simulink model "Copy_of_piddd"  (R2015b)
settings: Solver=VariableStepAuto  StartTime=0.0  StopTime=10.0  RelTol=1e-3
settings Model: Creator=ECPKn  LastModifiedBy=li

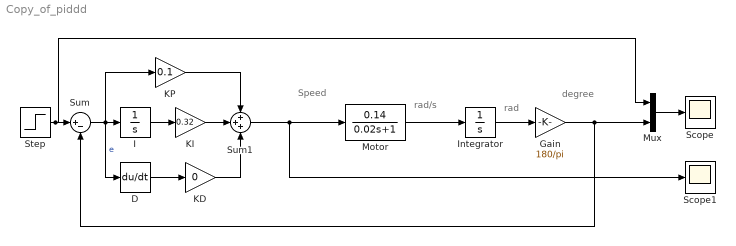
== system Copy_of_piddd ==
  note: degree
  note: rad
  note: rad/s
  note: Speed
  D : Derivative  CoefficientInTFapproximation=0.01
  Gain : Gain  Gain=180/pi
  I : Integrator
  Integrator : Integrator
  KD : Gain  Gain=0
  KI : Gain  Gain=0.32
  KP : Gain  Gain=0.1
  Motor : TransferFcn  Numerator=[0.14]  Denominator=[0.02 1]
  Mux : Mux  Inputs=2
  Scope : Scope
  Scope1 : Scope
  Step : Step  After=90  SampleTime=0
  Sum : Sum  Inputs=|+-
  Sum1 : Sum  Inputs=+++
  wires:
  Step/1 -> Mux/1, Sum/1
  Sum/1 -> KP/1, I/1, D/1  "e"
  Mux/1 -> Scope/1
  Gain/1 -> Mux/2, Sum/2
  Motor/1 -> Integrator/1
  Integrator/1 -> Gain/1
  D/1 -> KD/1
  Sum1/1 -> Scope1/1, Motor/1
  I/1 -> KI/1
  KI/1 -> Sum1/2
  KD/1 -> Sum1/3
  KP/1 -> Sum1/1
